simulink model "Lab4"  (R2012b)
settings: Solver=ode3  StartTime=0.0  StopTime=inf  FixedStep=0.015  RelTol=1e-3
settings Model: ExtModeTrigDuration=5000  Creator=runkunwang  LastModifiedBy=runkunwang
settings SolverCC: PositivePriorityOrder=on
settings RTWCC: SystemTargetFile=quarc_win64.tlc  TemplateMakefile=quarc_default_tmf  Description=QUARC Win64 Target  ProcessScript=quarc_win64_make_rtw_hook
settings STFCustomTargetCC: TargetPreCompLibLocation=C:\PROGRA~3\QUARC\lib\2012b\win64\release  CodeReplacementLibrary=ANSI_C  GeneratePreprocessorConditionals=Disable all  CombineOutputUpdateFcns=on  GRTInterface=off  SystemTargetFile=quarc_win64.tlc
settings GRTTargetCC: TargetPreCompLibLocation=C:\PROGRA~3\QUARC\lib\2012b\win64\release  ParMdlRefBuildCompliant=off  CompOptLevelCompliant=off  ConcurrentExecutionCompliant=off  MatFileLogging=off  ExtMode=on  ExtModeMexFile=quarc_comm

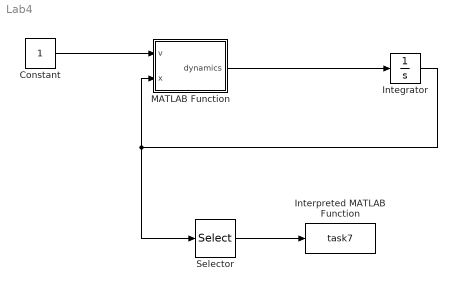
== system Lab4 ==
  Constant : Constant
  Integrator : Integrator  InitialCondition=[0;0;0;0]
  Interpreted MATLAB Function : MATLABFcn  MATLABFcn=task7  OutputDimensions=0
  MATLAB Function : MATLAB Function  TreatAsAtomicUnit=on
  Selector : Selector  InputPortWidth=4  IndexOptions=Index vector (dialog)  Indices=[1 3]  OutputSizes=1
  wires:
  MATLAB Function/1(dynamics) -> Integrator/1
  Integrator/1 -> Selector/1, MATLAB Function/2(x)
  Selector/1 -> Interpreted MATLAB Function/1
  Constant/1 -> MATLAB Function/1(v)

== matlab function Lab4/MATLAB Function ==
  data: v input; dynamics output; x input
function dynamics = fcn(v, x)
%#codegen
q1 = x(1);
q1d = x(2);
q2 = x(3);
q2d = x(4);

%t1 = (j1+m2*ladd^2)*(ra/(kt*kr));
%t2 = ((1/3)*m2*l2^2)*(ra/(kt*kr));
%t3 = (0.5*m2*ladd*l2)*(ra/(kt*kr));
%t4 = (m2*lc2)*(ra/(kt*kr));
%t5 = b1*(ra/(kt*kr))+kr*kv;
%t6 = b2*(ra/(kt*kr));

t1 = 0.0328869;
t2 = 0.0184263;
t3 = 0.0184263;
t4 = 0.0921317;
t5 = 0.6101446;
t6 = 0.0096726;

Cmat = [2*t2*sin(q2)*cos(q2)*q2d -t3*sin(q2)*q2d; -t2*sin(q2)*cos(q2)*q1d 0];
Mmat = [t1+t2*(sin(q2))^2 t3*cos(q2); t3*cos(q2) t2];
V = [v ; 0];
F = [t5*q1d ; t6*q2d];
G = [0 ; -t4*9.81*sin(q2)];

u = Mmat^(-1)*((V - Cmat*[q1d ; q2d]) - F - G);
xd = [q1d; u(1); q2d; u(2)];
dynamics = xd;
